simulink model "Lab2_1"  (Simulink 7.3)
settings: Solver=ode45  StartTime=0.0  StopTime=2.0  RelTol=1e-3
settings Model: Creator=Seva  LastModifiedBy=Seva

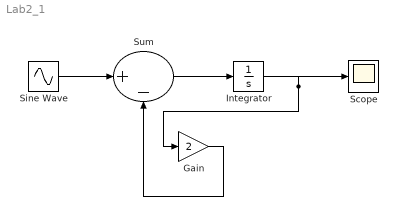
== system Lab2_1 ==
  Gain : Gain  Gain=2  ParameterDataTypeMode=double  ParameterDataType=fixdt(1, 16)  ParameterScaling=2^0  ParamDataTypeStr=double  OutDataTypeMode=double  OutDataTypeStr=double
  Integrator : Integrator
  Scope : Scope
  Sine Wave : Sin  Amplitude=1  Bias=0  Frequency=1  Phase=0  Samples=10  SampleTime=0  Offset=0
  Sum : Sum  Inputs=|+-  AccumDataTypeStr=double  OutDataTypeMode=double  OutDataTypeStr=double
  wires:
  Sum/1 -> Integrator/1
  Integrator/1 -> Gain/1, Scope/1
  Gain/1 -> Sum/2
  Sine Wave/1 -> Sum/1
